simulink model "state_feedback_cntrl"  (R2014a)
settings: Solver=ode3  StartTime=0.0  StopTime=6000*15  RelTol=1e-3
undefined symbols (not defined in the file): magnitude
libraries: aausat3_lib x20, hdlsllib x11, slrtlib x8, speedgoatlib_IO311 x5, dspmathops x1, simulink_extras x1
settings Model: BufferReuse=off  Creator=kasperv  LastModifiedBy=Aaltosatellites
settings SolverCC: EnableConcurrentExecution=on
settings DataIOCC: SignalLoggingSaveFormat=ModelDataLogs
settings OptimizationCC: BlockReduction=off  OptimizeBlockIOStorage=off  BufferReuse=off  GlobalBufferReuse=off  ExpressionFolding=off  ExpressionDepthLimit=2147483647  LocalBlockOutputs=off
settings DebuggingCC: UnderspecifiedInitializationDetection=Classic  FcnCallInpInsideContextMsg=UseLocalSettings  StateNameClashWarn=warning
settings HardwareCC: ProdIntDivRoundTo=Zero  ProdEndianess=LittleEndian  ProdHWDeviceType=Generic->32-bit x86 compatible
settings RTWCC: SystemTargetFile=slrt.tlc  TemplateMakefile=slrt_default_tmf  Description=Simulink Real-Time  ProcessScript=slrt_make_rtw_hook  RTWCompilerOptimization=On
settings SimulinkRealTimeCC: GeneratePreprocessorConditionals=Disable all  EnableShiftOperators=on

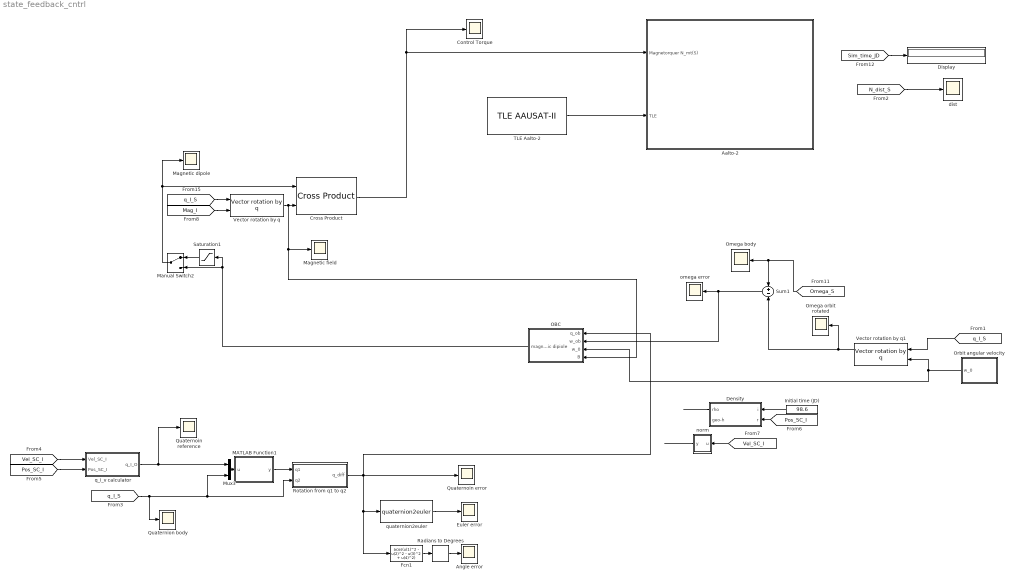
== system state_feedback_cntrl ==
  Aalto-2 : Subsystem  AncestorBlock=aausat3_lib/AAUSAT3  mask{r_com_s=[0.02 0.001 0.0], sat_temp_start=293.15, mass_sc=2.0, Dim=[0.207 0.1 0.1], inertia_c=[0.007,0.014,0.015], init_jd=2455153.1954318*0, q_s_c=[0 0 0 1], q_init_I_S=[0 1 0 0], w_init_s=[1,1,1]*0.2*(pi/180), Cd=2, rho=0.21850/1e12*0+9.9550/1e12*1+316.2/1e12*0, solar_m_flux=4.5565e-6, solar_absorb_coeff=1.5, theta_e=65, refldata=load('lib/AlbedoToolbox-1.0/refl_data/2005/ga050101-051231'), redfac=1, Ts=1, enable_sensor_emulation=on, enable_env_disturbance=on}
      mask prompts: r_com_s "Center of Mass:"; sat_temp_start "Start Temperature of the Satellite [K]:"; mass_sc "Mass of the Satellite [kg]:"; Dim "Satellite dimension"; inertia_c "Inertia Matrix of the Satellite:"; init_jd "Initial time [JD]:"; q_s_c "Controller Reference Frame (S->C):"; q_init_I_S "Initial Attitude (I->S):"; w_init_s "Initial Angular Rate (S) [rad/s]:"; Cd "Atmospheric Drag Coefficient [-]:"; rho "Atmospheric Density [kg/m^3]:"; solar_m_flux "Solar Momentum Flux [kg/ms^2]:"; solar_absorb_coeff "Solar Absorbtion Coefficient [-]:"; theta_e "Max. Angle of Theta [deg](eclipse: theta>r_earth/norm(R_SA)):"; refldata "Reflectivity Data (REFL Struct):"; redfac "Reduction Factor:"; Ts "Albedo Sampling Time [s]:"; enable_sensor_emulation "Enable Sensor Emulation."; enable_env_disturbance "Enable Environment Disturbance."
      mask Display:
      | image(imread('sat.jpg'));
      | color('w');
      | port_label('input', 1, 'N_mt(S)');
      | port_label('input', 2, 'TLE');
  Angle error : Scope
      settings: TimeRange=6000  YMin=0  YMax=85  SaveName=angle_error  SampleInput=on
  Control Torque : Scope
      settings: TimeRange=6000  YMin=-1.1e-05  YMax=1.1e-05  SaveName=control_torque  SampleInput=on
  Cross Product : aausat3_lib/Math Utilities/Vector operations/Cross Product
  Density : Subsystem
  Display : Display
  Euler error : Scope
      settings: TimeRange=6000  YMin=-3.5  YMax=3.5  SaveName=ScopeData3  SampleInput=on
  Fcn1 : Fcn  Expr=acos(u(1)^2 - u(2)^2 - u(3)^2 + u(4)^2)
  Initial time (JD) : Constant  Value=98.6
  MATLAB Function1 : MATLAB Function  TreatAsAtomicUnit=on
  Magnetic dipole : Scope
      settings: TimeRange=6000  YMin=-0.2  YMax=0.2  SaveName=magnetic_dipole  SampleInput=on
  Magnetic field : Scope
      settings: TimeRange=6000  YMin=-2.5e-05  YMax=2.5e-05  SaveName=magnetic_field  SampleInput=on
  Manual Switch2 : ManualSwitch
  Mux3 : Mux  Inputs=2
  OBC : Subsystem
  Omega body : Scope
      settings: TimeRange=6000  YMin=-0.55  YMax=0.55  SaveName=ScopeData6  SampleInput=on
  Omega orbit rotated : Scope
      settings: TimeRange=6000  YMin=-0.0011  YMax=0.0011  SaveName=ScopeData9  SampleInput=on
  Orbit angular velocity : Subsystem
  Quaternion body : Scope
      settings: TimeRange=6000  YMin=-1  YMax=1  SaveName=ScopeData8  SampleInput=on
  Quaternoin error : Scope
      settings: TimeRange=7000  YMin=-0.9  YMax=1  SaveName=quaternion_error  SampleInput=on
  Quaternoin reference : Scope
      settings: TimeRange=6000  YMin=-1  YMax=1  SampleInput=on
  Radians to Degrees : simulink_extras/Transformations/Radians to Degrees
  Rotation from q1 to q2 : Subsystem  AncestorBlock=aausat3_lib/Math Utilities/Quaternion operations/Rotation from q1 to q2
  Saturation1 : Saturate  UpperLimit=0.2  LowerLimit=-0.2
  Sum1 : Sum  Inputs=+-
  TLE Aalto-2 : aausat3_lib/Orbit and Ephemeris/TLE AAUSAT-II  satname='Aalto-2'  JulianDay=14321.69542252  xndt2o=0.00000555  xndd6o=0.0  bstar=.76898e-4  xincl=98.6  xnodeo=12.0  eo=0.002  omegao=254.1774  xmo=105.7862  xno=14.60096319131649561528*0+15.65129795862419730331*0+16.29879739439279729389*1  ts=1
  Vector rotation by q : aausat3_lib/Actuator Emulation/Permanent Magnet/Vector rotation by q
  Vector rotation by q1 : aausat3_lib/Math Utilities/Quaternion operations/Vector rotation by q
  dist : Scope
      settings: TimeRange=6000  YMin=-1e-05  YMax=1e-05  SaveName=dist  SampleInput=on
  norm : MATLAB Function  TreatAsAtomicUnit=on
  omega error : Scope
      settings: TimeRange=6000  YMin=-0.0012  YMax=0.0002  SaveName=angular_velocity  SampleInput=on
  q_i_v calculator : Subsystem
  quaternion2euler : aausat3_lib/Math Utilities/Quaternion operations/quaternion2euler
  wires:
  TLE Aalto-2/1 -> Aalto-2/2(TLE)
  [Sim_time_JD] -> Display/1
  [q_I_S] -> Vector rotation by q/1
  [Mag_I] -> Vector rotation by q/2
  OBC/1(magnetic dipiole) -> Saturation1/1, Manual Switch2/2
  Vector rotation by q/1 -> OBC/4(B), Magnetic field/1, Cross Product/2
  Saturation1/1 -> Manual Switch2/1
  Manual Switch2/1 -> Cross Product/1, Magnetic dipole/1
  [Pos_SC_I] -> q_i_v calculator/2(Pos_SC_I)
  [Vel_SC_I] -> q_i_v calculator/1(Vel_SC_I)
  Mux3/1 -> MATLAB Function1/1(u)
  [q_I_S] -> Quaternion body/1, Rotation from q1 to q2/2(q2), Mux3/2
  quaternion2euler/1 -> Euler error/1
  q_i_v calculator/1(q_I_O) -> Mux3/1, Quaternoin reference/1
  MATLAB Function1/1(y) -> Rotation from q1 to q2/1(q1)
  Fcn1/1 -> Radians to Degrees/1
  Radians to Degrees/1 -> Angle error/1
  Vector rotation by q1/1 -> Omega orbit rotated/1, Sum1/2
  [Omega_S] -> Sum1/1, Omega body/1
  Orbit angular velocity/1(w_0) -> OBC/3(w_0), Vector rotation by q1/2
  [q_I_S] -> Vector rotation by q1/1
  [N_dist_S] -> dist/1
  Cross Product/1 -> Aalto-2/1(Magnetorquer N_mt(S)), Control Torque/1
  Sum1/1 -> OBC/2(w_ob), omega error/1
  Rotation from q1 to q2/1(q_diff) -> OBC/1(q_ob), Quaternoin error/1, Fcn1/1, quaternion2euler/1
  Initial time (JD)/1 -> Density/1(i)
  Density/1(rho) -> ?
  norm/1(y) -> ?
  [Pos_SC_I] -> Density/2(r)
  [Vel_SC_I] -> norm/1(u)

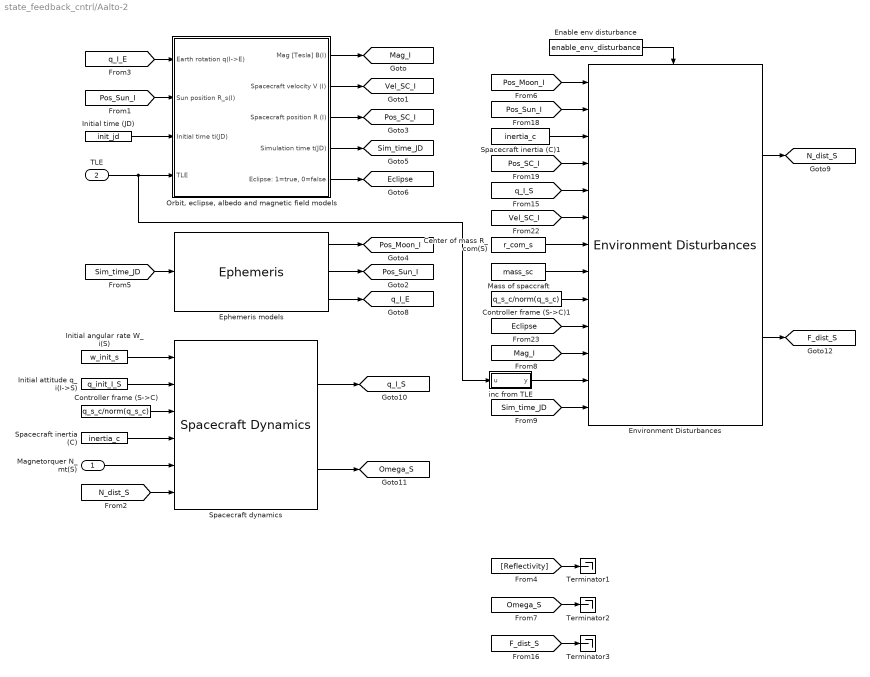
== system state_feedback_cntrl/Aalto-2 ==
  Magnetorquer N_mt(S) : Inport
  TLE : Inport  Port=2
  Center of mass R_com(S) : Constant  Value=r_com_s
  Controller frame (S->C) : Constant  Value=q_s_c/norm(q_s_c)
  Controller frame (S->C)1 : Constant  Value=q_s_c/norm(q_s_c)
  Enable env disturbance : Constant  Value=enable_env_disturbance
  Environment Disturbances : aausat3_lib/Disturbances/Environment Disturbances  Dim=Dim  sola_m_flux=solar_m_flux  solar_absorb_coeff=solar_absorb_coeff  rho=rho  Cd=Cd  G=6.672e-11  M_sun=1.989e30  M_earth=5.9742e24  M_moon=0.073483e24  enable_rad_dist=on  enable_atmospheric_dist=on  enable_gravity_dist=on  enable_mag_residual_dist=on
  Ephemeris models : aausat3_lib/Orbit and Ephemeris/Ephemeris
  Initial angular rate W_i(S) : Constant  Value=w_init_s
  Initial attitude q_i(I->S) : Constant  Value=q_init_I_S
  Initial time (JD) : Constant  Value=init_jd
  Mass of spaccraft : Constant  Value=mass_sc
  "Orbit, eclipse, albedo and magnetic field models" : Subsystem  AncestorBlock=aausat3_lib/Orbit and Ephemeris/Orbit and Magnetic field models  mask{theta_e=theta_e, refldata=refldata, redfac=redfac, Ts=Ts, r_e=6371e3, enable_eclipse=on, enable_IGRF=on, reflectivity_enabled=off, enable_sgp4=on, enable_custom_time=on}
      mask prompts: theta_e "Max. Angle of Theta [deg] (eclipse: theta > r_earth/norm(R_SA)):"; refldata "Reflectivity Data (REFL Struct):"; redfac "Reduction Factor:"; Ts "Albedo Model Sampling Time [s]:"; r_e "Radius of the Earth [m]:"; enable_eclipse "Enable Eclipse Model."; enable_IGRF "Enable IGRF Model."; reflectivity_enabled "Enable Albedo Model."; enable_sgp4 "Enable SGP4 Model."; enable_custom_time "Enable Custom Time."
      mask help: When you want to use "Other" make sure to define the TLE in the SGP4 subsystem.
  Spacecraft dynamics : aausat3_lib/Dynamics and Kinematics/Spacecraft Dynamics
  Spacecraft inertia (C) : Constant  Value=inertia_c
  Spacecraft inertia (C)1 : Constant  Value=inertia_c
  Terminator1 : Terminator
  Terminator2 : Terminator
  Terminator3 : Terminator
  inc from TLE : MATLAB Function  TreatAsAtomicUnit=on
  tag scope: Eclipse=global, F_dist_S=global, Mag_I=global, N_dist_S=global, Omega_S=global, Pos_Moon_I=global, Pos_SC_I=global, Pos_Sun_I=global, Sim_time_JD=global, Vel_SC_I=global, q_I_E=global, q_I_S=global
  wires:
  [q_I_S] -> Environment Disturbances/5
  Environment Disturbances/2 -> [F_dist_S]
  Environment Disturbances/1 -> [N_dist_S]
  [Mag_I] -> Environment Disturbances/11
  [Eclipse] -> Environment Disturbances/10
  Controller frame (S->C)1/1 -> Environment Disturbances/9
  Mass of spaccraft/1 -> Environment Disturbances/8
  Center of mass R_com(S)/1 -> Environment Disturbances/7
  [Vel_SC_I] -> Environment Disturbances/6
  [Pos_SC_I] -> Environment Disturbances/4
  Spacecraft inertia (C)1/1 -> Environment Disturbances/3
  [Pos_Sun_I] -> Environment Disturbances/2
  Enable env disturbance/1 -> Environment Disturbances/Enable
  [Pos_Moon_I] -> Environment Disturbances/1
  TLE/1 -> inc from TLE/1(u), "Orbit, eclipse, albedo and magnetic field models"/4(TLE)
  [q_I_E] -> "Orbit, eclipse, albedo and magnetic field models"/1(Earth rotation q(I->E))
  [Omega_S] -> Terminator2/1
  [Reflectivity] -> Terminator1/1
  Initial time (JD)/1 -> "Orbit, eclipse, albedo and magnetic field models"/3(Initial time ti(JD))
  [Pos_Sun_I] -> "Orbit, eclipse, albedo and magnetic field models"/2(Sun position R_s(I))
  Spacecraft dynamics/1 -> [q_I_S]
  [F_dist_S] -> Terminator3/1
  "Orbit, eclipse, albedo and magnetic field models"/5("Eclipse: 1=true, 0=false") -> [Eclipse]
  Magnetorquer N_mt(S)/1 -> Spacecraft dynamics/5
  "Orbit, eclipse, albedo and magnetic field models"/1(Mag [Tesla] B(I)) -> [Mag_I]
  "Orbit, eclipse, albedo and magnetic field models"/2(Spacecraft velocity V (I)) -> [Vel_SC_I]
  Spacecraft inertia (C)/1 -> Spacecraft dynamics/4
  Controller frame (S->C)/1 -> Spacecraft dynamics/3
  "Orbit, eclipse, albedo and magnetic field models"/3(Spacecraft position R (I)) -> [Pos_SC_I]
  Initial angular rate W_i(S)/1 -> Spacecraft dynamics/1
  Initial attitude q_i(I->S)/1 -> Spacecraft dynamics/2
  [Sim_time_JD] -> Environment Disturbances/13
  Ephemeris models/1 -> [Pos_Moon_I]
  Ephemeris models/2 -> [Pos_Sun_I]
  Ephemeris models/3 -> [q_I_E]
  Spacecraft dynamics/2 -> [Omega_S]
  [Sim_time_JD] -> Ephemeris models/1
  [N_dist_S] -> Spacecraft dynamics/6
  inc from TLE/1(y) -> Environment Disturbances/12
  "Orbit, eclipse, albedo and magnetic field models"/4(Simulation time t(JD)) -> [Sim_time_JD]

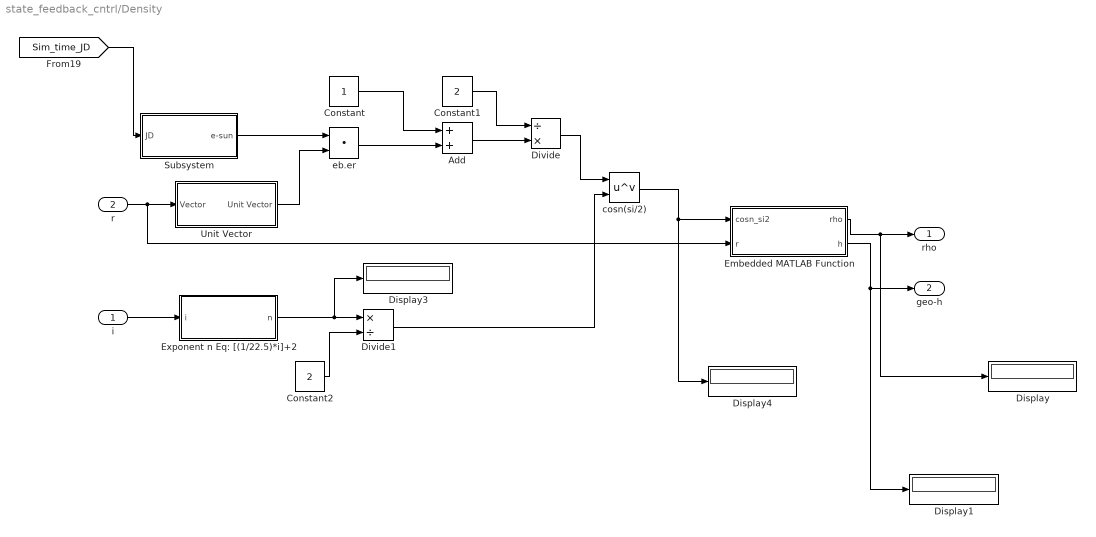
== system state_feedback_cntrl/Density ==
  i : Inport
  r : Inport  Port=2
  Add : Sum
  Constant : Constant
  Constant1 : Constant  Value=2
  Constant2 : Constant  Value=2
  Display{,1,3..4} (4 alike) : Display
  Divide : Product  Inputs=/*
  Divide1 : Product  Inputs=*/
  Embedded MATLAB Function : MATLAB Function  TreatAsAtomicUnit=on
  Exponent n Eq: [(1/22.5)*i]+2 : Subsystem
  Subsystem : Subsystem
  Unit Vector : Subsystem
  cosn(si/2) : Math  Operator=pow  SaturateOnIntegerOverflow=on
  eb.er : DotProduct  InputSameDT=on  OutDataTypeStr=Inherit: Inherit via internal rule
  rho : Outport
  geo-h : Outport  Port=2
  wires:
  r/1 -> Unit Vector/1(Vector), Embedded MATLAB Function/2(r)
  Unit Vector/1(Unit Vector) -> eb.er/2
  Constant/1 -> Add/1
  eb.er/1 -> Add/2
  Constant1/1 -> Divide/1
  Add/1 -> Divide/2
  i/1 -> Exponent n Eq: [(1/22.5)*i]+2/1(i)
  Exponent n Eq: [(1/22.5)*i]+2/1(n) -> Divide1/1, Display3/1
  Constant2/1 -> Divide1/2
  Divide/1 -> cosn(si/2)/1
  cosn(si/2)/1 -> Embedded MATLAB Function/1(cosn_si2), Display4/1
  Embedded MATLAB Function/1(rho) -> rho/1, Display/1
  Embedded MATLAB Function/2(h) -> Display1/1, geo-h/1
  Subsystem/1(e-sun) -> eb.er/1
  Divide1/1 -> cosn(si/2)/2
  [Sim_time_JD] -> Subsystem/1(JD)

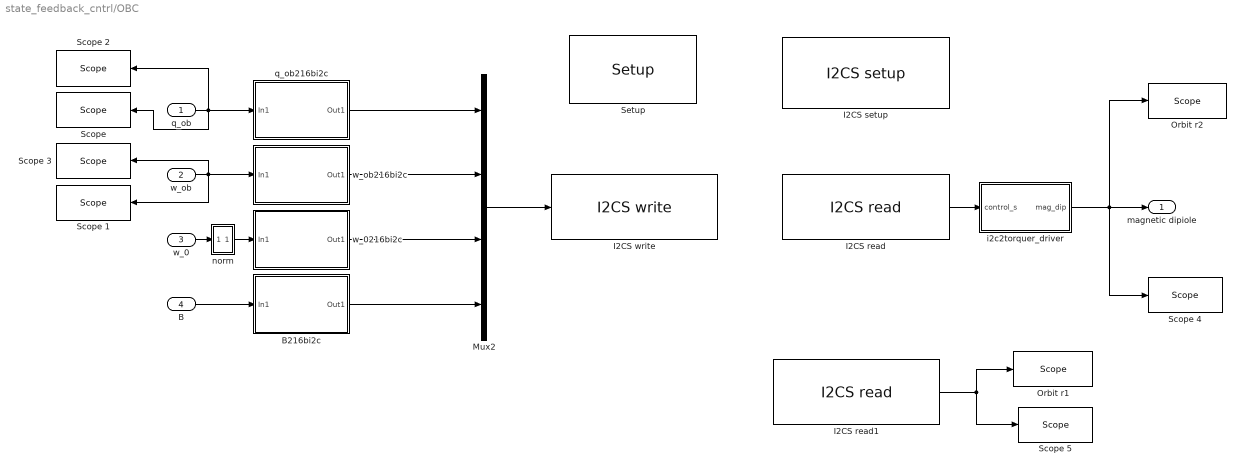
== system state_feedback_cntrl/OBC ==
  q_ob : Inport
  w_ob : Inport  Port=2
  w_0 : Inport  Port=3
  B : Inport  Port=4
  B216bi2c : Subsystem
  I2CS read : speedgoatlib_IO311/I2C/I2CS read  id=1  chan=1  regs=[1 2 3]  ts=0.001  pciSlot=-1
  I2CS read1 : speedgoatlib_IO311/I2C/I2CS read  id=1  chan=1  regs=[26 27 28 29]  ts=0.001  pciSlot=-1
  I2CS setup : speedgoatlib_IO311/I2C/I2CS setup  id=1  chan=1  slaveID=4  ts=-1  pciSlot=-1
  I2CS write : speedgoatlib_IO311/I2C/I2CS write  id=1  chan=1  regs=[4 5 6 7 8 9 10 11 12 13 14 15 16 17 18 19 20 21 22 23 24 25]  ts=0.001  pciSlot=-1
  Mux2 : Mux
  Orbit r1 : slrtlib/Displays and Logging/Scope   scopeno=9  scopetype=File  autostart=on  viewmode=Numerical  formatstr='%15.6f'  grid=on  ylimits=[0,0]  nosamples=1000000  noprepostsamples=0  interleave=100  triggermode=FreeRun  triggersignal=1  trigsignalfromport=off  triggerlevel=0.0  triggerslope=Either  triggerscope=1  triggersample=0  filename=timings1.dat  mode=Lazy  writesize=512*1024*1024  autorestart=off  dynamicfilemode=off  maxwritefilesize=512*1024^2
  Orbit r2 : slrtlib/Displays and Logging/Scope   scopeno=7  scopetype=File  autostart=on  viewmode=Numerical  formatstr='%15.6f'  grid=on  ylimits=[0,0]  nosamples=10000000  noprepostsamples=0  interleave=10  triggermode=Scope triggering  triggersignal=1  trigsignalfromport=off  triggerlevel=0.0  triggerslope=Either  triggerscope=1  triggersample=0  filename=dipole_m.dat  mode=Lazy  writesize=512*1024*1024  autorestart=off  dynamicfilemode=off  maxwritefilesize=512*1024^2
  "Scope " : slrtlib/Displays and Logging/Scope   scopeno=5  scopetype=File  autostart=on  viewmode=Graphical redraw  formatstr='%15.6f'  grid=on  ylimits=[0,0]  nosamples=100000  noprepostsamples=0  interleave=1000  triggermode=FreeRun  triggersignal=1  trigsignalfromport=off  triggerlevel=0.0  triggerslope=Either  triggerscope=1  triggersample=0  filename=q_ob1.dat  mode=Lazy  writesize=512*1024  autorestart=off  dynamicfilemode=off  maxwritefilesize=512*1024^2
  Scope 1 : slrtlib/Displays and Logging/Scope   scopeno=1  scopetype=File  autostart=on  viewmode=Graphical redraw  formatstr='%15.6f'  grid=on  ylimits=[0,0]  nosamples=100000  noprepostsamples=0  interleave=1000  triggermode=FreeRun  triggersignal=1  trigsignalfromport=off  triggerlevel=0.0  triggerslope=Either  triggerscope=1  triggersample=0  filename=w_ob1.dat  mode=Lazy  writesize=512*1024  autorestart=off  dynamicfilemode=off  maxwritefilesize=512*1024^2
  Scope 2 : slrtlib/Displays and Logging/Scope   scopeno=2  scopetype=Target  autostart=on  viewmode=Graphical sliding  formatstr='%15.6f'  grid=on  ylimits=[0,0]  nosamples=1000  noprepostsamples=0  interleave=1000  triggermode=FreeRun  triggersignal=1  trigsignalfromport=off  triggerlevel=0.0  triggerslope=Either  triggerscope=1  triggersample=0  filename=q_ob1.dat  mode=Lazy  writesize=512*1024  autorestart=off  dynamicfilemode=off  maxwritefilesize=512*1024^2
  Scope 3 : slrtlib/Displays and Logging/Scope   scopeno=3  scopetype=Target  autostart=on  viewmode=Graphical sliding  formatstr='%15.6f'  grid=on  ylimits=[0,0]  nosamples=1000  noprepostsamples=0  interleave=1000  triggermode=FreeRun  triggersignal=1  trigsignalfromport=off  triggerlevel=0.0  triggerslope=Either  triggerscope=1  triggersample=0  filename=w_ob1.dat  mode=Lazy  writesize=512*1024  autorestart=off  dynamicfilemode=off  maxwritefilesize=512*1024^2
  Scope 4 : slrtlib/Displays and Logging/Scope   scopeno=4  scopetype=Target  autostart=on  viewmode=Graphical sliding  formatstr='%15.6f'  grid=on  ylimits=[0,0]  nosamples=100000  noprepostsamples=0  interleave=10  triggermode=FreeRun  triggersignal=1  trigsignalfromport=off  triggerlevel=0.0  triggerslope=Either  triggerscope=1  triggersample=0  filename=w_ob1.dat  mode=Lazy  writesize=512*1024  autorestart=off  dynamicfilemode=off  maxwritefilesize=512*1024^2
  Scope 5 : slrtlib/Displays and Logging/Scope   scopeno=6  scopetype=Target  autostart=on  viewmode=Graphical sliding  formatstr='%15.6f'  grid=on  ylimits=[0,0]  nosamples=1000  noprepostsamples=0  interleave=1000  triggermode=FreeRun  triggersignal=1  trigsignalfromport=off  triggerlevel=0.0  triggerslope=Either  triggerscope=1  triggersample=0  filename=w_ob1.dat  mode=Lazy  writesize=512*1024  autorestart=off  dynamicfilemode=off  maxwritefilesize=512*1024^2
  Setup : speedgoatlib_IO311/Setup/Setup  group=Lower channel group setup  id=1  fpga1=speedgoat_IO311_CI_01264  pciSlot=-1  lowerDirection=[1, 1, 0, 0, 1, 0, 1, 0, 0, 0, 0, 0, 0, 0, 0, 0]  lowerReset=[1]  lowerValue=[0]  upperDirection=[0, 0, 0, 0, 0, 0, 0, 0, 0, 0, 0, 0, 0, 0, 0, 0]  upperReset=[1]  upperValue=[0]
  i2c2torquer_driver : Subsystem
  norm : MATLAB Function  TreatAsAtomicUnit=on
  q_ob216bi2c : Subsystem
  w_0216bi2c : Subsystem
  w_ob216bi2c : Subsystem
  magnetic dipiole : Outport
  wires:
  Mux2/1 -> I2CS write/1
  I2CS read/1 -> i2c2torquer_driver/1(control_s)
  B/1 -> B216bi2c/1(In1)
  i2c2torquer_driver/1(mag_dip) -> Scope 4/1, Orbit r2/1, magnetic dipiole/1
  w_ob/1 -> Scope 3/1, w_ob216bi2c/1(In1), Scope 1/1
  q_ob/1 -> Scope 2/1, q_ob216bi2c/1(In1), "Scope "/1
  w_0/1 -> norm/1(u)
  norm/1(y) -> w_0216bi2c/1(In1)
  q_ob216bi2c/1(Out1) -> Mux2/1
  w_ob216bi2c/1(Out1) -> Mux2/2
  w_0216bi2c/1(Out1) -> Mux2/3
  B216bi2c/1(Out1) -> Mux2/4
  I2CS read1/1 -> Scope 5/1, Orbit r1/1

== system state_feedback_cntrl/Orbit angular velocity ==
  Cross Product1 : aausat3_lib/Math Utilities/Vector operations/Cross Product
  Normalization : dspmathops/Normalization  NormType=Squared 2-norm  Bias=1e-10  NormOver=Each column  ColComp=on  Dimension=1  outputDataTypeStr=Inherit: Same as product output  outputLastDataTypeStr=Inherit: Same as product output  outputMin=[]  outputMax=[]  accumDataTypeStr=Inherit: Same as product output  accumLastDataTypeStr=Inherit: Same as product output  roundingMode=Floor  overflowMode=off
  w_0 : Outport
  wires:
  Cross Product1/1 -> w_0/1
  [Vel_SC_I] -> Cross Product1/2
  [Pos_SC_I] -> Normalization/1
  Normalization/1 -> Cross Product1/1

== system state_feedback_cntrl/Rotation from q1 to q2 ==
  q1 : Inport
  q2 : Inport  Port=2
  Quaternion inverter : Subsystem
  Quaternion mulitiplication : S-Function  FunctionName=qmul  EnableBusSupport=off
  q_diff : Outport
  wires:
  q1/1 -> Quaternion inverter/1(q)
  Quaternion inverter/1(q^-1) -> Quaternion mulitiplication/1
  q2/1 -> Quaternion mulitiplication/2
  Quaternion mulitiplication/1 -> q_diff/1

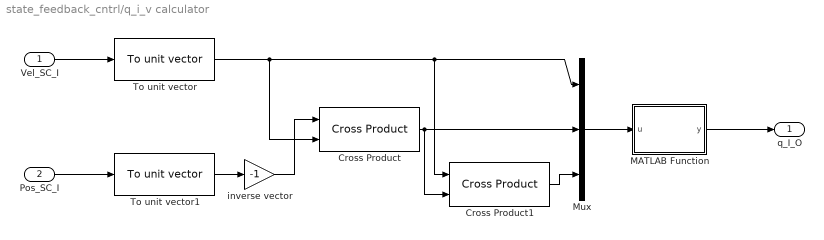
== system state_feedback_cntrl/q_i_v calculator ==
  Vel_SC_I : Inport
  Pos_SC_I : Inport  Port=2
  Cross Product : aausat3_lib/Math Utilities/Vector operations/Cross Product
  Cross Product1 : aausat3_lib/Math Utilities/Vector operations/Cross Product
  MATLAB Function : MATLAB Function  TreatAsAtomicUnit=on
  Mux : Mux  Inputs=3
  To unit vector : aausat3_lib/Math Utilities/Vector operations/To unit vector
  To unit vector1 : aausat3_lib/Math Utilities/Vector operations/To unit vector
  inverse vector : Gain  Gain=-1
  q_I_O : Outport
  wires:
  MATLAB Function/1(y) -> q_I_O/1
  Pos_SC_I/1 -> To unit vector1/1
  Vel_SC_I/1 -> To unit vector/1
  To unit vector/1 -> Cross Product/2, Mux/1, Cross Product1/1
  inverse vector/1 -> Cross Product/1
  To unit vector1/1 -> inverse vector/1
  Mux/1 -> MATLAB Function/1(u)
  Cross Product/1 -> Mux/2, Cross Product1/2
  Cross Product1/1 -> Mux/3

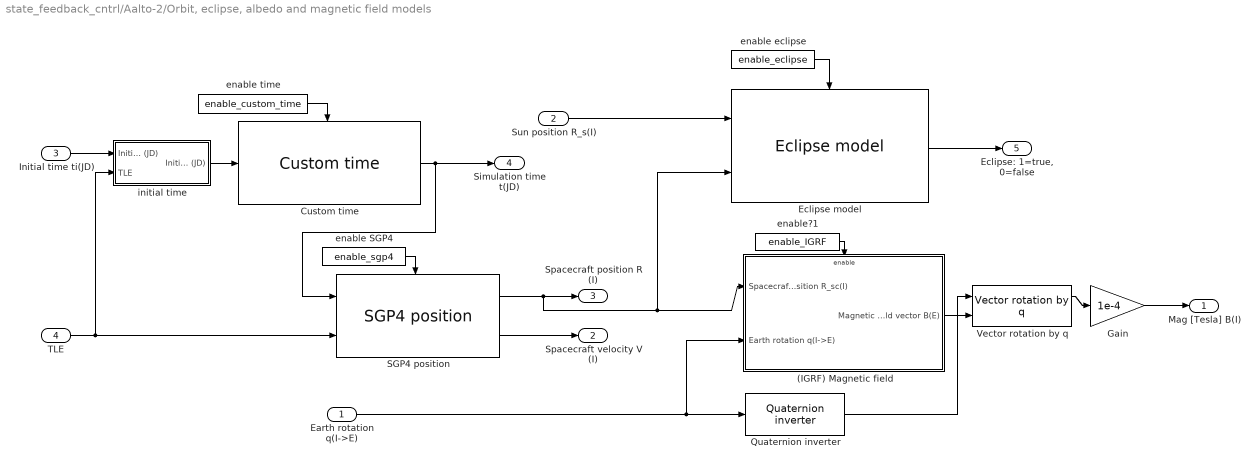
== system state_feedback_cntrl/Aalto-2/Orbit, eclipse, albedo and magnetic field models ==
  Earth rotation q(I->E) : Inport
  Sun position R_s(I) : Inport  Port=2
  Initial time ti(JD) : Inport  Port=3
  TLE : Inport  Port=4
  (IGRF) Magnetic field : Subsystem  AncestorBlock=aausat3_lib/Orbit and Ephemeris/(IGRF) Magnetic field  TreatAsAtomicUnit=on
  Custom time : aausat3_lib/Orbit and Ephemeris/Custom time
  Eclipse model : aausat3_lib/Orbit and Ephemeris/Eclipse model  r_e=r_e  enable=off  theta_e=theta_e
  Gain : Gain  Gain=1e-4
  Quaternion inverter : aausat3_lib/Math Utilities/Quaternion operations/Quaternion inverter
  SGP4 position : aausat3_lib/Orbit and Ephemeris/SGP4 position
  Vector rotation by q : aausat3_lib/Math Utilities/Quaternion operations/Vector rotation by q
  enable SGP4 : Constant  Value=enable_sgp4
  enable eclipse : Constant  Value=enable_eclipse
  enable time : Constant  Value=enable_custom_time
  enable?1 : Constant  Value=enable_IGRF
  initial time : Subsystem
  Mag [Tesla] B(I) : Outport
  Spacecraft velocity V (I) : Outport  Port=2
  Spacecraft position R (I) : Outport  Port=3
  Simulation time t(JD) : Outport  Port=4
  "Eclipse: 1=true, 0=false" : Outport  Port=5  PortDimensions=1
  wires:
  Initial time ti(JD)/1 -> initial time/1(Initial time in (JD))
  initial time/1(Initial time out (JD)) -> Custom time/1
  TLE/1 -> initial time/2(TLE), SGP4 position/2
  enable eclipse/1 -> Eclipse model/Enable
  Gain/1 -> Mag [Tesla] B(I)/1
  (IGRF) Magnetic field/1(Magnetic field vector B(E)) -> Vector rotation by q/2
  SGP4 position/2 -> Spacecraft velocity V (I)/1
  SGP4 position/1 -> Spacecraft position R (I)/1, Eclipse model/2, (IGRF) Magnetic field/1(Spacecraft position R_sc(I))
  enable SGP4/1 -> SGP4 position/Enable
  Earth rotation q(I->E)/1 -> Quaternion inverter/1, (IGRF) Magnetic field/2(Earth rotation q(I->E))
  Sun position R_s(I)/1 -> Eclipse model/1
  Custom time/1 -> SGP4 position/1, Simulation time t(JD)/1
  enable time/1 -> Custom time/Enable
  Quaternion inverter/1 -> Vector rotation by q/1
  Vector rotation by q/1 -> Gain/1
  enable?1/1 -> (IGRF) Magnetic field/Enable
  Eclipse model/1 -> "Eclipse: 1=true, 0=false"/1

== system state_feedback_cntrl/Density/Exponent n Eq: [(1//22.5)*i]+2 ==
  i : Inport
  Add : Sum
  Product : Product  RndMeth=Zero
  a : Constant  Value=1/22.5
  b : Constant  Value=2
  n : Outport
  wires:
  a/1 -> Product/2
  Product/1 -> Add/1
  b/1 -> Add/2
  i/1 -> Product/1
  Add/1 -> n/1

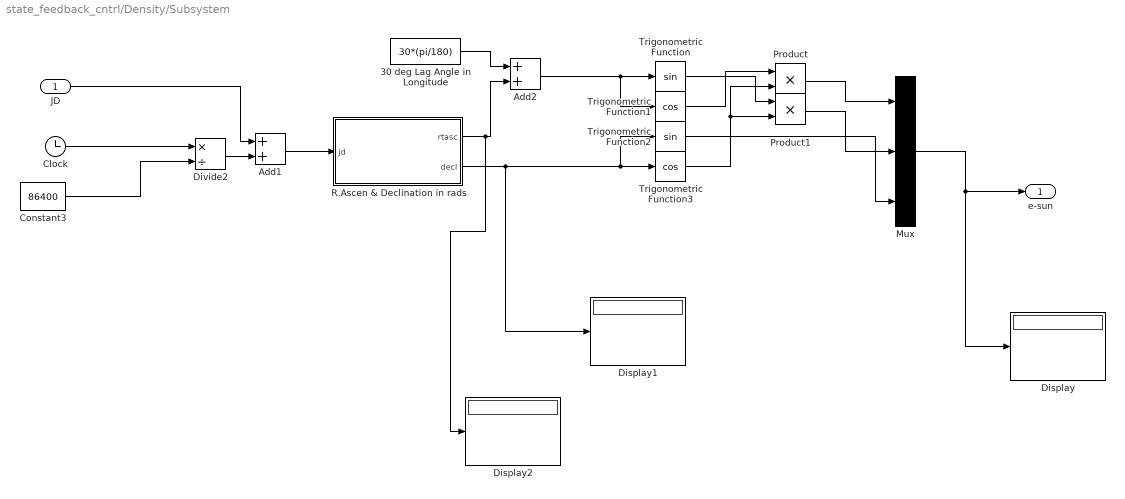
== system state_feedback_cntrl/Density/Subsystem ==
  JD : Inport
  30 deg Lag Angle in Longitude : Constant  Value=30*(pi/180)
  Add1 : Sum
  Add2 : Sum
  Clock : Clock
  Constant3 : Constant  Value=86400
  Display : Display
  Display1 : Display
  Display2 : Display
  Divide2 : Product  Inputs=*/
  Mux : Mux  Inputs=3
  Product : Product  RndMeth=Zero
  Product1 : Product  RndMeth=Zero
  R.Ascen & Declination in rads : MATLAB Function  TreatAsAtomicUnit=on
  Trigonometric Function : Trigonometry
  Trigonometric Function1 : Trigonometry  Operator=cos
  Trigonometric Function2 : Trigonometry
  Trigonometric Function3 : Trigonometry  Operator=cos
  e-sun : Outport
  wires:
  Clock/1 -> Divide2/1
  Constant3/1 -> Divide2/2
  Divide2/1 -> Add1/2
  JD/1 -> Add1/1
  Add1/1 -> R.Ascen & Declination in rads/1(jd)
  30 deg Lag Angle in Longitude/1 -> Add2/1
  R.Ascen & Declination in rads/1(rtasc) -> Add2/2, Display2/1
  Add2/1 -> Trigonometric Function/1, Trigonometric Function1/1
  R.Ascen & Declination in rads/2(decl) -> Display1/1, Trigonometric Function3/1, Trigonometric Function2/1
  Trigonometric Function1/1 -> Product/1
  Trigonometric Function3/1 -> Product/2, Product1/2
  Trigonometric Function/1 -> Product1/1
  Product/1 -> Mux/1
  Product1/1 -> Mux/2
  Trigonometric Function2/1 -> Mux/3
  Mux/1 -> e-sun/1, Display/1

== system state_feedback_cntrl/Density/Unit Vector ==
  Vector : Inport
  Divide1 : Product  Inputs=*/
  Vector Mag : Subsystem
  Unit Vector : Outport
  wires:
  Vector Mag/1(Magnitude) -> Divide1/2
  Vector/1 -> Divide1/1, Vector Mag/1(Vector)
  Divide1/1 -> Unit Vector/1

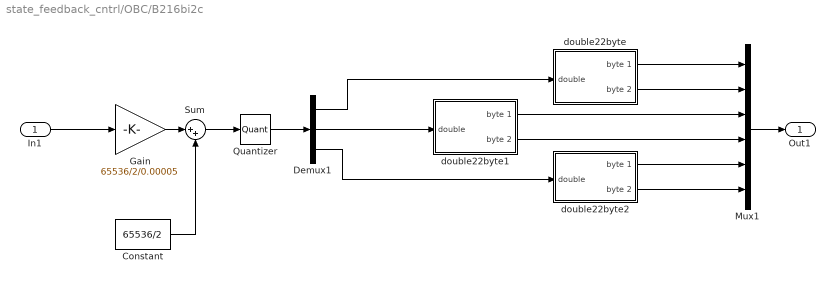
== system state_feedback_cntrl/OBC/B216bi2c ==
  In1 : Inport
  Constant : Constant  Value=65536/2  SampleTime=-1
  Demux1 : Demux  Outputs=3
  Gain : Gain  Gain=65536/2/0.00005
  Mux1 : Mux  Inputs=6
  Quantizer : Quantizer  QuantizationInterval=1
  Sum : Sum  Inputs=|++
  double22byte : Subsystem
  double22byte1 : Subsystem
  double22byte2 : Subsystem
  Out1 : Outport
  wires:
  double22byte1/1(byte 1) -> Mux1/3
  double22byte1/2(byte 2) -> Mux1/4
  Mux1/1 -> Out1/1
  Constant/1 -> Sum/2
  Sum/1 -> Quantizer/1
  Gain/1 -> Sum/1
  Demux1/2 -> double22byte1/1(double)
  Demux1/3 -> double22byte2/1(double)
  Quantizer/1 -> Demux1/1
  double22byte2/1(byte 1) -> Mux1/5
  In1/1 -> Gain/1
  double22byte2/2(byte 2) -> Mux1/6
  Demux1/1 -> double22byte/1(double)
  double22byte/1(byte 1) -> Mux1/1
  double22byte/2(byte 2) -> Mux1/2

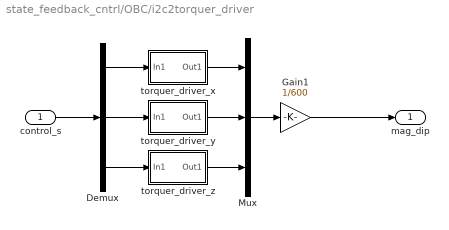
== system state_feedback_cntrl/OBC/i2c2torquer_driver ==
  control_s : Inport
  Demux : Demux  Outputs=3
  Gain1 : Gain  Gain=1/600
  Mux : Mux  Inputs=3
  torquer_driver_x : Subsystem
  torquer_driver_y : Subsystem
  torquer_driver_z : Subsystem
  mag_dip : Outport
  wires:
  Demux/2 -> torquer_driver_y/1(In1)
  Gain1/1 -> mag_dip/1
  Demux/3 -> torquer_driver_z/1(In1)
  torquer_driver_z/1(Out1) -> Mux/3
  torquer_driver_y/1(Out1) -> Mux/2
  Mux/1 -> Gain1/1
  control_s/1 -> Demux/1
  Demux/1 -> torquer_driver_x/1(In1)
  torquer_driver_x/1(Out1) -> Mux/1

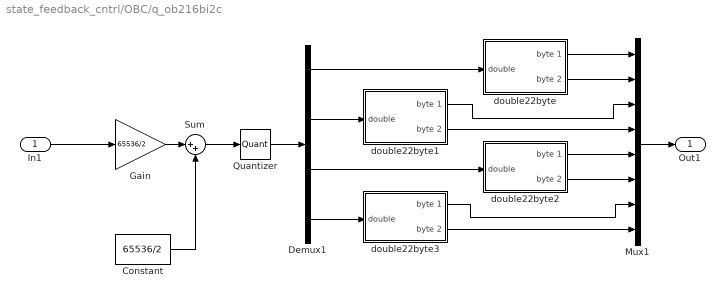
== system state_feedback_cntrl/OBC/q_ob216bi2c ==
  In1 : Inport
  Constant : Constant  Value=65536/2
  Demux1 : Demux
  Gain : Gain  Gain=65536/2
  Mux1 : Mux  Inputs=8
  Quantizer : Quantizer  QuantizationInterval=1
  Sum : Sum  Inputs=|++
  double22byte : Subsystem
  double22byte1 : Subsystem
  double22byte2 : Subsystem
  double22byte3 : Subsystem
  Out1 : Outport
  wires:
  double22byte1/1(byte 1) -> Mux1/3
  double22byte1/2(byte 2) -> Mux1/4
  Mux1/1 -> Out1/1
  Constant/1 -> Sum/2
  Sum/1 -> Quantizer/1
  Gain/1 -> Sum/1
  Demux1/2 -> double22byte1/1(double)
  Demux1/3 -> double22byte2/1(double)
  Quantizer/1 -> Demux1/1
  double22byte2/1(byte 1) -> Mux1/5
  In1/1 -> Gain/1
  double22byte2/2(byte 2) -> Mux1/6
  Demux1/1 -> double22byte/1(double)
  double22byte/1(byte 1) -> Mux1/1
  double22byte/2(byte 2) -> Mux1/2
  Demux1/4 -> double22byte3/1(double)
  double22byte3/1(byte 1) -> Mux1/7
  double22byte3/2(byte 2) -> Mux1/8

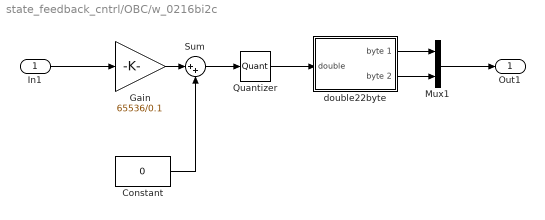
== system state_feedback_cntrl/OBC/w_0216bi2c ==
  In1 : Inport
  Constant : Constant  Value=0
  Gain : Gain  Gain=65536/0.1
  Mux1 : Mux  Inputs=2
  Quantizer : Quantizer  QuantizationInterval=1
  Sum : Sum  Inputs=|++
  double22byte : Subsystem
  Out1 : Outport
  wires:
  Mux1/1 -> Out1/1
  Constant/1 -> Sum/2
  Sum/1 -> Quantizer/1
  Gain/1 -> Sum/1
  In1/1 -> Gain/1
  Quantizer/1 -> double22byte/1(double)
  double22byte/1(byte 1) -> Mux1/1
  double22byte/2(byte 2) -> Mux1/2

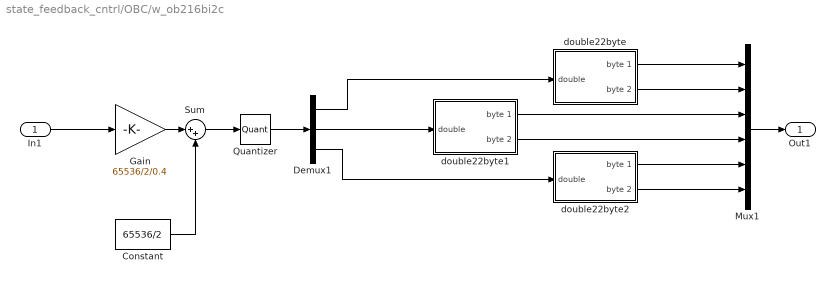
== system state_feedback_cntrl/OBC/w_ob216bi2c ==
  In1 : Inport
  Constant : Constant  Value=65536/2
  Demux1 : Demux  Outputs=3
  Gain : Gain  Gain=65536/2/0.4
  Mux1 : Mux  Inputs=6
  Quantizer : Quantizer  QuantizationInterval=1
  Sum : Sum  Inputs=|++
  double22byte : Subsystem
  double22byte1 : Subsystem
  double22byte2 : Subsystem
  Out1 : Outport
  wires:
  double22byte1/1(byte 1) -> Mux1/3
  double22byte1/2(byte 2) -> Mux1/4
  Mux1/1 -> Out1/1
  Constant/1 -> Sum/2
  Sum/1 -> Quantizer/1
  Gain/1 -> Sum/1
  Demux1/2 -> double22byte1/1(double)
  Demux1/3 -> double22byte2/1(double)
  Quantizer/1 -> Demux1/1
  double22byte2/1(byte 1) -> Mux1/5
  In1/1 -> Gain/1
  double22byte2/2(byte 2) -> Mux1/6
  Demux1/1 -> double22byte/1(double)
  double22byte/1(byte 1) -> Mux1/1
  double22byte/2(byte 2) -> Mux1/2

== system state_feedback_cntrl/Rotation from q1 to q2/Quaternion inverter ==
  q : Inport
  Demux : Demux
  Demux1 : Demux  Outputs=3
  Gain : Gain  Gain=-1  SaturateOnIntegerOverflow=on  OutDataTypeStr=Inherit: Same as input  ParamDataTypeStr=Inherit: Same as input
  Mux : Mux
  Mux1 : Mux  Inputs=3
  q^-1 : Outport
  wires:
  q/1 -> Demux/1
  Mux/1 -> q^-1/1
  Demux/4 -> Mux/4
  Demux/1 -> Mux1/1
  Demux/2 -> Mux1/2
  Demux/3 -> Mux1/3
  Mux1/1 -> Gain/1
  Demux1/1 -> Mux/1
  Demux1/2 -> Mux/2
  Demux1/3 -> Mux/3
  Gain/1 -> Demux1/1

== system state_feedback_cntrl/Aalto-2/Orbit, eclipse, albedo and magnetic field models/(IGRF) Magnetic field ==
  Spacecraft position R_sc(I) : Inport
  Earth rotation q(I->E) : Inport  Port=2
  Enable : EnablePort
  Magnetic field model : Subsystem
  T->Gauss : Gain  Gain=1e4  SaturateOnIntegerOverflow=on  OutDataTypeStr=Inherit: Same as input  ParamDataTypeStr=Inherit: Same as input
  Vector rotation by q : aausat3_lib/Math Utilities/Quaternion operations/Vector rotation by q
  Magnetic field vector B(E) : Outport
  wires:
  Spacecraft position R_sc(I)/1 -> Vector rotation by q/2
  Earth rotation q(I->E)/1 -> Vector rotation by q/1
  Vector rotation by q/1 -> Magnetic field model/1(R_sc(E))
  Magnetic field model/1(B(E)) -> T->Gauss/1  "B(I / E)"
  T->Gauss/1 -> Magnetic field vector B(E)/1

== system state_feedback_cntrl/Aalto-2/Orbit, eclipse, albedo and magnetic field models/initial time ==
  Initial time in (JD) : Inport
  TLE : Inport  Port=2
  Demux : Demux  Outputs=12
  Mux1 : Mux  Inputs=12
  Switch : Switch  Criteria=u2 > Threshold
  "TLE -> JD converter" : aausat3_lib/Other Model Utilities/TLE -> JD converter
  Terminator : Terminator
  Initial time out (JD) : Outport
  wires:
  Mux1/1 -> Terminator/1
  Switch/1 -> Initial time out (JD)/1
  Initial time in (JD)/1 -> Switch/1, Switch/2
  TLE/1 -> Demux/1
  Demux/2 -> Mux1/2
  Demux/3 -> Mux1/3
  Demux/4 -> Mux1/4
  Demux/5 -> Mux1/5
  Demux/6 -> Mux1/6
  Demux/7 -> Mux1/7
  Demux/8 -> Mux1/8
  Demux/9 -> Mux1/9
  Demux/10 -> Mux1/10
  Demux/11 -> Mux1/11
  Demux/12 -> Mux1/12
  Demux/1 -> "TLE -> JD converter"/1
  "TLE -> JD converter"/1 -> Switch/3, Mux1/1

== system state_feedback_cntrl/Density/Unit Vector/Vector Mag ==
  Vector : Inport
  Demux : Demux  Outputs=3
  Math Function : Math  Operator=magnitude^2  SaturateOnIntegerOverflow=on
  Math Function1 : Math  Operator=sqrt  SaturateOnIntegerOverflow=on
  Sum : Sum  Inputs=+++
  Magnitude : Outport
  wires:
  Math Function/1 -> Demux/1
  Demux/1 -> Sum/1
  Demux/2 -> Sum/2
  Demux/3 -> Sum/3
  Sum/1 -> Math Function1/1
  Math Function1/1 -> Magnitude/1
  Vector/1 -> Math Function/1

== system state_feedback_cntrl/OBC/B216bi2c/double22byte ==
  double : Inport
  Bit Shift : hdlsllib/HDL Operations/Bit Shift  mode=Shift Right Arithmetic  N=8
  Constant2 : Constant  Value=256
  Product : Product
  Rounding Function : Rounding
  Sum4 : Sum  Inputs=-+|
  byte 1 : Outport
  byte 2 : Outport  Port=2
  wires:
  double/1 -> Sum4/2, Bit Shift/1
  Bit Shift/1 -> Rounding Function/1
  Sum4/1 -> byte 2/1
  Constant2/1 -> Product/1
  Product/1 -> Sum4/1
  Rounding Function/1 -> byte 1/1, Product/2

== system state_feedback_cntrl/OBC/B216bi2c/double22byte1 ==
  double : Inport
  Bit Shift : hdlsllib/HDL Operations/Bit Shift  mode=Shift Right Arithmetic  N=8
  Constant2 : Constant  Value=256
  Product : Product
  Rounding Function : Rounding
  Sum4 : Sum  Inputs=-+|
  byte 1 : Outport
  byte 2 : Outport  Port=2
  wires:
  double/1 -> Sum4/2, Bit Shift/1
  Bit Shift/1 -> Rounding Function/1
  Sum4/1 -> byte 2/1
  Constant2/1 -> Product/1
  Product/1 -> Sum4/1
  Rounding Function/1 -> byte 1/1, Product/2

== system state_feedback_cntrl/OBC/B216bi2c/double22byte2 ==
  double : Inport
  Bit Shift : hdlsllib/HDL Operations/Bit Shift  mode=Shift Right Arithmetic  N=8
  Constant2 : Constant  Value=256
  Product : Product
  Rounding Function : Rounding
  Sum4 : Sum  Inputs=-+|
  byte 1 : Outport
  byte 2 : Outport  Port=2
  wires:
  double/1 -> Sum4/2, Bit Shift/1
  Bit Shift/1 -> Rounding Function/1
  Sum4/1 -> byte 2/1
  Constant2/1 -> Product/1
  Product/1 -> Sum4/1
  Rounding Function/1 -> byte 1/1, Product/2

== system state_feedback_cntrl/OBC/i2c2torquer_driver/torquer_driver_x ==
  In1 : Inport
  Constant1 : Constant  Value=256
  Sum1 : Sum  Inputs=|-+
  Switch : Switch  Criteria=u2 > Threshold  Threshold=128
  Out1 : Outport
  wires:
  In1/1 -> Sum1/2, Switch/2, Switch/3
  Constant1/1 -> Sum1/1
  Sum1/1 -> Switch/1
  Switch/1 -> Out1/1

== system state_feedback_cntrl/OBC/i2c2torquer_driver/torquer_driver_y ==
  In1 : Inport
  Constant1 : Constant  Value=256
  Sum1 : Sum  Inputs=|-+
  Switch : Switch  Criteria=u2 > Threshold  Threshold=128
  Out1 : Outport
  wires:
  In1/1 -> Sum1/2, Switch/2, Switch/3
  Constant1/1 -> Sum1/1
  Sum1/1 -> Switch/1
  Switch/1 -> Out1/1

== system state_feedback_cntrl/OBC/i2c2torquer_driver/torquer_driver_z ==
  In1 : Inport
  Constant1 : Constant  Value=256
  Sum1 : Sum  Inputs=|-+
  Switch : Switch  Criteria=u2 > Threshold  Threshold=128
  Out1 : Outport
  wires:
  In1/1 -> Sum1/2, Switch/2, Switch/3
  Constant1/1 -> Sum1/1
  Sum1/1 -> Switch/1
  Switch/1 -> Out1/1

== system state_feedback_cntrl/OBC/q_ob216bi2c/double22byte ==
  double : Inport
  Bit Shift : hdlsllib/HDL Operations/Bit Shift  mode=Shift Right Arithmetic  N=8
  Constant2 : Constant  Value=256
  Product : Product
  Rounding Function : Rounding
  Sum4 : Sum  Inputs=-+|
  byte 1 : Outport
  byte 2 : Outport  Port=2
  wires:
  double/1 -> Sum4/2, Bit Shift/1
  Bit Shift/1 -> Rounding Function/1
  Sum4/1 -> byte 2/1
  Constant2/1 -> Product/1
  Product/1 -> Sum4/1
  Rounding Function/1 -> byte 1/1, Product/2

== system state_feedback_cntrl/OBC/q_ob216bi2c/double22byte1 ==
  double : Inport
  Bit Shift : hdlsllib/HDL Operations/Bit Shift  mode=Shift Right Arithmetic  N=8
  Constant2 : Constant  Value=256
  Product : Product
  Rounding Function : Rounding
  Sum4 : Sum  Inputs=-+|
  byte 1 : Outport
  byte 2 : Outport  Port=2
  wires:
  double/1 -> Sum4/2, Bit Shift/1
  Bit Shift/1 -> Rounding Function/1
  Sum4/1 -> byte 2/1
  Constant2/1 -> Product/1
  Product/1 -> Sum4/1
  Rounding Function/1 -> byte 1/1, Product/2

== system state_feedback_cntrl/OBC/q_ob216bi2c/double22byte2 ==
  double : Inport
  Bit Shift : hdlsllib/HDL Operations/Bit Shift  mode=Shift Right Arithmetic  N=8
  Constant2 : Constant  Value=256
  Product : Product
  Rounding Function : Rounding
  Sum4 : Sum  Inputs=-+|
  byte 1 : Outport
  byte 2 : Outport  Port=2
  wires:
  double/1 -> Sum4/2, Bit Shift/1
  Bit Shift/1 -> Rounding Function/1
  Sum4/1 -> byte 2/1
  Constant2/1 -> Product/1
  Product/1 -> Sum4/1
  Rounding Function/1 -> byte 1/1, Product/2

== system state_feedback_cntrl/OBC/q_ob216bi2c/double22byte3 ==
  double : Inport
  Bit Shift : hdlsllib/HDL Operations/Bit Shift  mode=Shift Right Arithmetic  N=8
  Constant2 : Constant  Value=256
  Product : Product
  Rounding Function : Rounding
  Sum4 : Sum  Inputs=-+|
  byte 1 : Outport
  byte 2 : Outport  Port=2
  wires:
  double/1 -> Sum4/2, Bit Shift/1
  Bit Shift/1 -> Rounding Function/1
  Sum4/1 -> byte 2/1
  Constant2/1 -> Product/1
  Product/1 -> Sum4/1
  Rounding Function/1 -> byte 1/1, Product/2

== system state_feedback_cntrl/OBC/w_0216bi2c/double22byte ==
  double : Inport
  Bit Shift : hdlsllib/HDL Operations/Bit Shift  mode=Shift Right Arithmetic  N=8
  Constant2 : Constant  Value=256
  Product : Product
  Rounding Function : Rounding
  Sum4 : Sum  Inputs=-+|
  byte 1 : Outport
  byte 2 : Outport  Port=2
  wires:
  double/1 -> Sum4/2, Bit Shift/1
  Bit Shift/1 -> Rounding Function/1
  Sum4/1 -> byte 2/1
  Constant2/1 -> Product/1
  Product/1 -> Sum4/1
  Rounding Function/1 -> byte 1/1, Product/2

== system state_feedback_cntrl/OBC/w_ob216bi2c/double22byte ==
  double : Inport
  Bit Shift : hdlsllib/HDL Operations/Bit Shift  mode=Shift Right Arithmetic  N=8
  Constant2 : Constant  Value=256
  Product : Product
  Rounding Function : Rounding
  Sum4 : Sum  Inputs=-+|
  byte 1 : Outport
  byte 2 : Outport  Port=2
  wires:
  double/1 -> Sum4/2, Bit Shift/1
  Bit Shift/1 -> Rounding Function/1
  Sum4/1 -> byte 2/1
  Constant2/1 -> Product/1
  Product/1 -> Sum4/1
  Rounding Function/1 -> byte 1/1, Product/2

== system state_feedback_cntrl/OBC/w_ob216bi2c/double22byte1 ==
  double : Inport
  Bit Shift : hdlsllib/HDL Operations/Bit Shift  mode=Shift Right Arithmetic  N=8
  Constant2 : Constant  Value=256
  Product : Product
  Rounding Function : Rounding
  Sum4 : Sum  Inputs=-+|
  byte 1 : Outport
  byte 2 : Outport  Port=2
  wires:
  double/1 -> Sum4/2, Bit Shift/1
  Bit Shift/1 -> Rounding Function/1
  Sum4/1 -> byte 2/1
  Constant2/1 -> Product/1
  Product/1 -> Sum4/1
  Rounding Function/1 -> byte 1/1, Product/2

== system state_feedback_cntrl/OBC/w_ob216bi2c/double22byte2 ==
  double : Inport
  Bit Shift : hdlsllib/HDL Operations/Bit Shift  mode=Shift Right Arithmetic  N=8
  Constant2 : Constant  Value=256
  Product : Product
  Rounding Function : Rounding
  Sum4 : Sum  Inputs=-+|
  byte 1 : Outport
  byte 2 : Outport  Port=2
  wires:
  double/1 -> Sum4/2, Bit Shift/1
  Bit Shift/1 -> Rounding Function/1
  Sum4/1 -> byte 2/1
  Constant2/1 -> Product/1
  Product/1 -> Sum4/1
  Rounding Function/1 -> byte 1/1, Product/2

== system state_feedback_cntrl/Aalto-2/Orbit, eclipse, albedo and magnetic field models/(IGRF) Magnetic field/Magnetic field model ==
  R_sc(E) : Inport
  S-Function : S-Function  FunctionName=igrfS2  Parameters=2009,13  EnableBusSupport=off
  B(E) : Outport
  wires:
  S-Function/1 -> B(E)/1
  R_sc(E)/1 -> S-Function/1

== matlab function state_feedback_cntrl/MATLAB Function1 ==
  data: u input; y output
function y = fcn(u)
     q = u(1:4);
     p = u(5:8);
     y = [q_pick_near(p', q')']; 
     
end

== matlab function state_feedback_cntrl/OBC/norm ==
  data: u input; y output
function y = fcn(u)
%#codegen

y = norm(u);

== matlab function state_feedback_cntrl/q_i_v calculator/MATLAB Function ==
  data: u input; y output
function y = fcn(u)
%#codegen

y = dcmatrix_and_q(u);

== matlab function state_feedback_cntrl/Aalto-2/inc from TLE ==
  data: u input; y output
function y = fcn(u)
%#codegen

y = u(7);

== matlab function state_feedback_cntrl/Density/Embedded MATLAB Function ==
  data: cosn_si2 input; r input; rho output; h output
function [rho,h] = Density(cosn_si2,r)

ellipsoid = [6378.137e3, 0.081819190842];
x = r(1);
y = r(2);
z = r(3);

Csi=cosn_si2; %Cosn(si/2)
%************************************************************
%Formula taken from ecef2geodetic function of Matlab
% Ellipsoid constants
a  = ellipsoid(1);       % Semimajor axis
e2 = ellipsoid(2) ^ 2;   % Square of first eccentricity
ep2 = e2 / (1 - e2);     % Square of second eccentricity
f = 1 - sqrt(1 - e2);    % Flattening
b = a * (1 - f);         % Semiminor axis

% Longitude
lambda = atan2(y,x);

% Distance from Z-axis
rho = hypot(x,y);

% Bowring's formula for initial parametric (beta) and geodetic (phi) latitudes
beta = atan2(z, (1 - f) * rho);
phi = atan2(z   + b * ep2 * sin(beta).^3,...
            rho - a * e2  * cos(beta).^3);

% Fixed-point iteration with Bowring's formula
% (typically converges within two or three iterations)
betaNew = atan2((1 - f)*sin(phi), cos(phi));
count = 0;
while any(beta(:) ~= betaNew(:)) && count < 5
    beta = betaNew;
    phi = atan2(z   + b * ep2 * sin(beta).^3,...
                rho - a * e2  * cos(beta).^3);
    betaNew = atan2((1 - f)*sin(phi), cos(phi));
    count = count + 1;
end

% Calculate ellipsoidal height from the final value for latitude
sinphi = sin(phi);
N = a ./ sqrt(1 - e2 * sinphi.^2);
h = rho .* cos(phi) + (z + e2 * N .* sinphi) .* sinphi - N;
%*************************************************************************
h=h/1000;%in Km

%% Harris-Priester Density Table
% h(km), rho-min(g/km3), rho-max(g/km3))
HP = [100, 497400, 497400; ...
    120, 24900, 24900; ...
    130, 8377, 8710; ...
    140, 3899, 4059; ...
    150, 2122, 2215; ...
    160, 1263, 1344; ...
    170, 800.80, 875.80; ...
    180, 528.30, 601; ...
    190, 361.70, 429.70; ...
    200, 255.70, 316.20; ...
    210, 183.90, 239.60; ...
    220, 134.10, 185.30; ...
    230, 99.490, 145.50; ...
    240, 74.880, 115.70; ...
    250, 57.090, 93.080; ...
    260, 44.030, 75.550; ...
    270, 34.300, 61.820; ...
    280, 26.970, 50.950; ...
    290, 21.390, 42.260; ...
    300, 17.080, 35.260; ...
    320, 10.990, 25.110; ...
    340, 7.2140, 18.190; ...
    360, 4.8240, 13.370; ...
    380, 3.2740, 9.9550; ...
    400, 2.2490, 7.4920; ...
    420, 1.5580, 5.6840; ...
    440, 1.0910, 4.3550; ...
    460, 0.77010, 3.3620; ...
    480, 0.54740, 2.6120; ...
    500, 0.39160, 2.0420; ...
    520, 0.28190, 1.6050; ...
    540, 0.20420, 1.2670; ...
    560, 0.14880, 1.0050; ...
    580, 0.10920, 0.79970; ...
    600, 0.080700, 0.63900; ...
    620, 0.060120, 0.51230; ...
    640, 0.045190, 0.41210; ...
    660, 0.034300, 0.33250; ...
    680, 0.026320, 0.26910; ...
    700, 0.020430, 0.21850; ...
    720, 0.016070, 0.17790; ...
    740, 0.012810, 0.14520; ...
    760, 0.010360, 0.11900; ...
    780, 0.0084960, 0.097760; ...
    800, 0.0070690, 0.080590; ...
    840, 0.0046800, 0.057410; ...
    880, 0.0032000, 0.042100; ...
    920, 0.0022100, 0.031300; ...
    960, 0.0015600, 0.023600; ...
    1000, 0.0011500, 0.018100];
%%
if h>HP(end,1)
    error('Too high altitude');
    rho=0;
elseif h<HP(1,1)
    error('Too low altitude');
    rho=0;
else
    indxi=find(HP(:,1)<=h);
    hi=HP(indxi(end),1);
    rho_m_i=HP(indxi(end),2);
    rho_M_i=HP(indxi(end),3);
    
    indxii=find(HP(:,1)>=h);
    hii=HP(indxii(1),1);
    rho_m_ii=HP(indxii(1),2);
    rho_M_ii=HP(indxii(1),3);
    
    Hm=(hi-hii)/log(rho_m_ii/rho_m_i);
    HM=(hi-hii)/log(rho_M_ii/rho_M_i);
    
    rho_m=rho_m_i*exp((hi-h)/Hm);
    rho_M=rho_M_i*exp((hi-h)/HM);
    
    rho=rho_m+((rho_M-rho_m)*Csi);
    rho=rho/1e12; %in Kg/m3
end

== matlab function state_feedback_cntrl/Density/Subsystem/R.Ascen & Declination in rads ==
  data: jd input; rtasc output; decl output
function [rtasc,decl] = sun ( jd )

        twopi      =     2.0*pi;
        deg2rad    =     pi/180.0;

        % -------------------------  implementation   -----------------
        % -------------------  initialize values   --------------------
        tut1= ( jd - 2451545.0  )/ 36525.0;
%fprintf(1,'tut1 %14.9f \n',tut1);

        meanlong= 280.460  + 36000.77*tut1;
        meanlong= rem( meanlong,360.0  );  %deg

        ttdb= tut1;
        meananomaly= 357.5277233  + 35999.05034 *ttdb;
        meananomaly= rem( meananomaly*deg2rad,twopi );  %rad
        if ( meananomaly < 0.0  )
            meananomaly= twopi + meananomaly;
          end

        eclplong= meanlong + 1.914666471 *sin(meananomaly) ...
                    + 0.019994643 *sin(2.0 *meananomaly); %deg

        obliquity= 23.439291  - 0.0130042 *ttdb;  %deg

        meanlong = meanlong*deg2rad;
        if ( meanlong < 0.0  )
            meanlong= twopi + meanlong;
          end
        eclplong = eclplong *deg2rad;
        obliquity= obliquity *deg2rad;

        % --------- find magnitude of sun vector, )   components ------
        magr= 1.000140612  - 0.016708617 *cos( meananomaly ) ...
                              - 0.000139589 *cos( 2.0 *meananomaly );    % in au's

%         rsun(1)= magr*cos( eclplong );
%         rsun(2)= magr*cos(obliquity)*sin(eclplong);
%         rsun(3)= magr*sin(obliquity)*sin(eclplong);

%fprintf(1,'meanlon %11.6f meanan %11.6f eclplon %11.6f obli %11.6f \n', ...
           %meanlong/deg2rad,meananomaly/deg2rad,(2.0*pi+eclplong)/deg2rad,obliquity/deg2rad);
%fprintf(1,'rs %11.9f %11.9f %11.9f \n',rsun);
%fprintf(1,'magr %14.7f \n',magr);
%%%%rsun
%%%%rsun*149597870.0

        rtasc= atan( cos(obliquity)*tan(eclplong) );

        % --- check that rtasc is in the same quadrant as eclplong ----
        if ( eclplong < 0.0  )
            eclplong= eclplong + twopi;    % make sure it's in 0 to 2pi range
          end
        if ( abs( eclplong-rtasc ) > pi*0.5  )
            rtasc= rtasc + 0.5 *pi*round( (eclplong-rtasc)/(0.5 *pi));
          end
%fprintf(1,'rtasc %11.6f \n',rtasc/deg2rad);
        decl = asin( sin(obliquity)*sin(eclplong) );
%fprintf(1,'decl %11.6f \n',decl/deg2rad);

== matlab function state_feedback_cntrl/norm ==
  data: u input; y output
function y = fcn(u)
%#codegen

y = norm(u);
